simulink model "RobotPitcherFinal"  (R2015a)
settings: Solver=ode4  StartTime=0.0  StopTime=20  FixedStep=.01  RelTol=1e-3
settings Model: Creator=jesseweisberg  LastModifiedBy=jesseweisberg
settings ModelReferenceCC: EnableParallelModelReferenceBuilds=on  ParallelModelReferenceMATLABWorkerInit=Copy Base Workspace

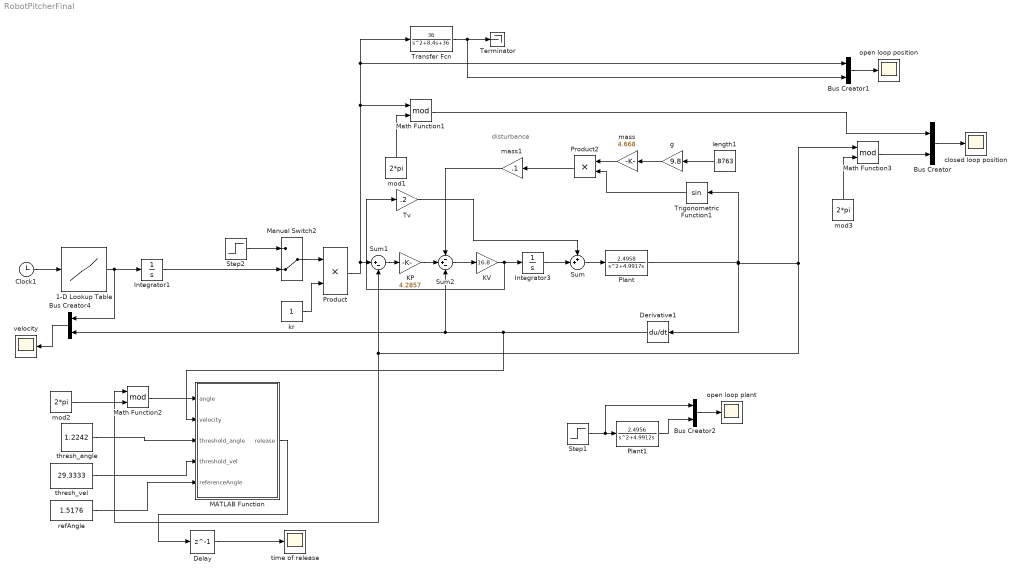
== system RobotPitcherFinal ==
  note: disturbance
  1-D Lookup Table : Lookup_n-D  NumberOfTableDimensions=1  BreakpointsForDimension1=[0, 3, 15, 16,20]  Table=[0, 29.33, 29.33, 0, 0]  RndMeth=Simplest  InputSameDT=on
  Bus Creator{,1..2,4} (4 alike) : BusCreator  Inputs=2
  Clock1 : Clock
  Delay : Delay  DelayLength=1  InitialCondition=0
  Derivative1 : Derivative
  Integrator1 : Integrator
  Integrator3 : Integrator
  KP : Gain  Gain=4.2857
  KV : Gain  Gain=16.8
  MATLAB Function : MATLAB Function  TreatAsAtomicUnit=on
  Manual Switch2 : ManualSwitch  CurrentSetting=0
  Math Function1 : Math  Operator=mod  SaturateOnIntegerOverflow=on
  Math Function2 : Math  Operator=mod  SaturateOnIntegerOverflow=on
  Math Function3 : Math  Operator=mod  SaturateOnIntegerOverflow=on
  Plant : TransferFcn  Numerator=[2.4958]  Denominator=[1 4.9917 0]
  Plant1 : TransferFcn  Numerator=[2.4956]  Denominator=[1 4.9912 0]
  Product : Product
  Product2 : Product
  Step1 : Step  After=10  SampleTime=0
  Step2 : Step  After=10  SampleTime=0
  Sum : Sum  Inputs=++|
  Sum1 : Sum  Inputs=|+-
  Sum2 : Sum  Inputs=-+-
  Terminator : Terminator
  Transfer Fcn : TransferFcn  Numerator=[36]  Denominator=[1 8.4 36]
  Trigonometric Function1 : Trigonometry
  Tv : Gain  Gain=.2
  closed loop position : Scope
      settings: TimeRange=5  YMin=0  YMax=1  SaveName=closedLoop_system
  g : Gain  Gain=9.8
  kr : Constant
  "length1 " : Constant  Value=.8763
  mass : Gain  Gain=4.668
  mass1 : Gain  Gain=.1
  mod1 : Constant  Value=2*pi
  mod2 : Constant  Value=2*pi
  mod3 : Constant  Value=2*pi
  open loop plant : Scope
      settings: YMin=-0.575  YMax=-0.2  SaveName=stepResponse_manipulator
  open loop position : Scope
      settings: YMin=-0.559062  YMax=-0.505818  SaveName=openloop_system
  refAngle : Constant  Value=1.5176
  thresh_angle : Constant  Value=1.2242
  thresh_vel : Constant  Value=29.3333
  time of release : Scope
      settings: YMin=-0.575  YMax=-0.2  SaveName=timeRelease
  velocity : Scope
      settings: YMin=-2.5  YMax=40  SaveName=velocityTrajectoryResponse
  wires:
  KV/1 -> Integrator3/1, Tv/1
  Tv/1 -> Sum/1
  Sum1/1 -> KP/1
  Sum2/1 -> KV/1
  Bus Creator/1 -> closed loop position/1
  1-D Lookup Table/1 -> Bus Creator4/1, Integrator1/1
  Integrator3/1 -> Sum/2
  kr/1 -> Product/2
  Transfer Fcn/1 -> Terminator/1, Bus Creator1/2
  Product/1 -> Sum1/1, Math Function1/1, Transfer Fcn/1, Bus Creator1/1
  Bus Creator1/1 -> open loop position/1
  Bus Creator2/1 -> open loop plant/1
  Sum/1 -> Plant/1
  Step1/1 -> Bus Creator2/1, Plant1/1
  Clock1/1 -> 1-D Lookup Table/1
  Bus Creator4/1 -> velocity/1
  Step2/1 -> Manual Switch2/1
  Manual Switch2/1 -> Product/1
  KP/1 -> Sum2/2
  mass1/1 -> Sum2/1
  Plant1/1 -> Bus Creator2/2
  Integrator1/1 -> Manual Switch2/2
  thresh_angle/1 -> MATLAB Function/3(threshold_angle)
  thresh_vel/1 -> MATLAB Function/4(threshold_vel)
  MATLAB Function/1(release) -> Delay/1
  Delay/1 -> time of release/1
  refAngle/1 -> MATLAB Function/5(referenceAngle)
  Math Function2/1 -> MATLAB Function/1(angle)
  mod2/1 -> Math Function2/2
  Plant/1 -> Trigonometric Function1/1, Math Function2/1, Sum1/2, Math Function3/1, Derivative1/1
  mod3/1 -> Math Function3/2
  g/1 -> mass/1
  "length1 "/1 -> g/1
  mass/1 -> Product2/1
  Trigonometric Function1/1 -> Product2/2
  Product2/1 -> mass1/1
  Math Function3/1 -> Bus Creator/2
  mod1/1 -> Math Function1/2
  Math Function1/1 -> Bus Creator/1
  Derivative1/1 -> Bus Creator4/2, Sum2/3, MATLAB Function/2(velocity)

== matlab function RobotPitcherFinal/MATLAB Function ==
  data: angle input; release output; velocity input; threshold_angle input; threshold_vel input; referenceAngle input
function release = fcn(angle, velocity, threshold_angle,threshold_vel, referenceAngle)
%#codegen
 
if (angle >= threshold_angle && angle<=referenceAngle && velocity >= threshold_vel)
release=1;
else
release=0;
end
